simulink model "pmsm_foc_drive"  (R2026a)
settings: Solver=ode4  StopTime=5  FixedStep=1e-6
undefined symbols (not defined in the file): D, I_max, J, Ki_i, Ki_w, Kp_i, Kp_w, L, P, phi_m, Rs, T_s, Tpwm, V_max, Vdc
libraries: simulink x6, slpidlib x4, sl_discontinuities x1
settings Model: Creator=Lemão Som  LastModifiedBy=Lemão Som

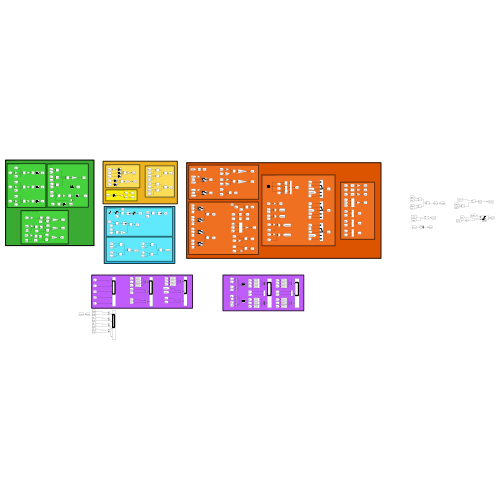
[thumbnail: Simulink's stored preview of the top-level diagram]
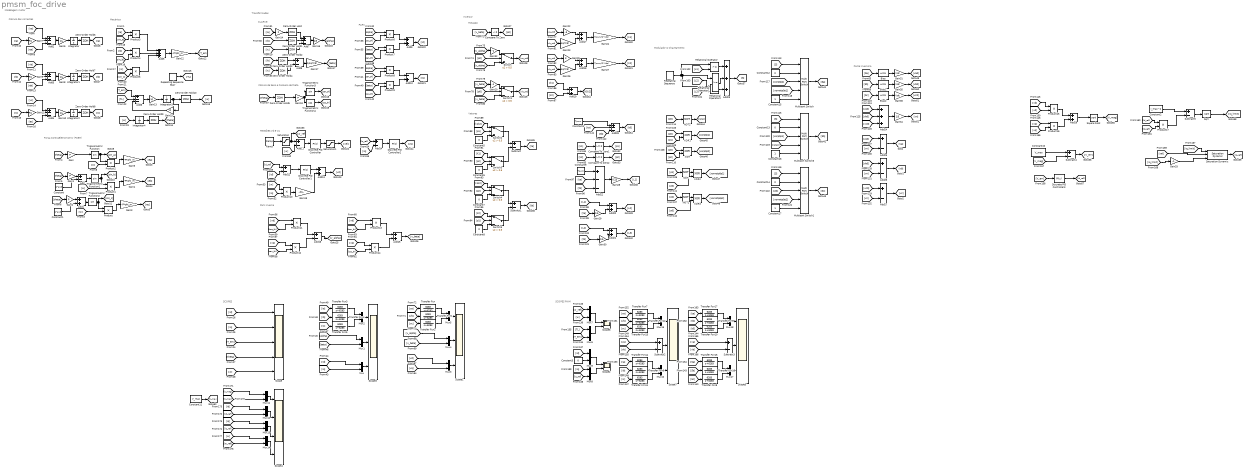
== system pmsm_foc_drive ==
  note: Ponte Inversora
  note: Modulador & Chaveamento
  note: Vetores
  note: Rotação
  note: SCOPES
  note: Cálculo de Seno e Cosseno de theta
  note: Transformadas
  note: Modelagem motor
  note: Inversor
  note: Park Inversa
  note: TENSÕES Vd E Vq
  note: PARK
  note: CLARKE
  note: Mecânica
  note: Força ContraEletromotriz (FCEM)
  note: Cálculo das correntes
  note: SCOPES PWM
  Add{,8,11..12,14,16,25..27} (9 alike) : Sum  Inputs=+-
  Add{1,9,13,15,17..21,29} (10 alike) : Sum
  Add10 : Sum  Inputs=-+
  Add{2..4,6..7,22,28} (7 alike) : Sum  Inputs=+--
  Add23 : Sum  Inputs=+++
  Add24 : Sum  Inputs=+++
  Add5 : Sum  Inputs=+++
  Bias : Bias  Bias=-0.5  SaturateOnIntegerOverflow=off
  Bias1 : Bias  Bias=-0.5  SaturateOnIntegerOverflow=off
  Bias2 : Bias  Bias=-0.5  SaturateOnIntegerOverflow=off
  Compare To Zero : simulink/Logic and Bit Operations/Compare To Zero  relop=<  OutDataTypeStr=boolean
  Compare To Zero1 : simulink/Logic and Bit Operations/Compare To Zero  relop=>=  OutDataTypeStr=boolean  ZeroCross=off
  Compare To Zero2 : simulink/Logic and Bit Operations/Compare To Zero  relop=>=  OutDataTypeStr=boolean  ZeroCross=off
  Constant : Constant  Value=2*pi/3
  Constant1 : Constant  Value=2*pi/3
  Constant10 : Constant  Value=V_max
  Constant11 : Constant  Value=V_max
  Constant{3,5..8,12..14} (8 alike) : Constant  Value=0
  Constant15 : Constant
  Constant16 : Constant
  Constant17 : Constant
  Constant2 : Constant  Value=I_max^2
  Constant4 : Constant  Value=Tpwm  VectorParams1D=off
  Constant9 : Constant  Value=Tpwm
  Discrete PID Controller : slpidlib/PID Controller  Controller=PI  Form=Parallel  TimeDomain=Discrete-time  UseExternalTs=off  SampleTime=T_s  IntegratorMethod=Forward Euler  FilterMethod=Forward Euler  ControllerParametersSource=internal  P=Kp_w  I=Ki_w  UseKiTs=off  D=0  UseExternalDerivativeSource=off  N=100  UseFilter=on  TunerSelectOption=Transfer Function Based (PID Tuner App)  InitialConditionSource=internal  InitialConditionForIntegrator=0  InitialConditionForFilter=0  DifferentiatorICPrevScaledInput=0  ExternalReset=none  TrackingMode=off  Kt=1  LimitOutput=on  SatLimitsSource=internal  UpperSaturationLimit=100  LowerSaturationLimit=-100  LinearizeAsGain=off  AntiWindupMode=clamping  Kb=1  LimitIntegrator=off  UpperIntegratorSaturationLimit=inf  LowerIntegratorSaturationLimit=-inf  POutMin=[]  POutMax=[]  IOutMin=[]  IOutMax=[]  DOutMin=[]  DOutMax=[]  NOutMin=[]  NOutMax=[]  SumOutMin=[]  SumOutMax=[]  SaturationOutMin=[]  SaturationOutMax=[]  PParamMin=[]  PParamMax=[]  IParamMin=[]  IParamMax=[]  DParamMin=[]  DParamMax=[]  NParamMin=[]  NParamMax=[]  KbParamMin=[]  KbParamMax=[]  KtParamMin=[]  KtParamMax=[]  KbOutMin=[]  KbOutMax=[]  KtOutMin=[]  KtOutMax=[]  IntegratorOutMin=[]  IntegratorOutMax=[]  FilterOutMin=[]  FilterOutMax=[]  SumI1OutMin=[]  SumI1OutMax=[]  SumI2OutMin=[]  SumI2OutMax=[]  SumI3OutMin=[]  SumI3OutMax=[]  SumI4OutMin=[]  SumI4OutMax=[]  SumDOutMin=[]  SumDOutMax=[]  DifferentiatorOutMin=[]  DifferentiatorOutMax=[]  FilterDiffOutCoefMin=[]  FilterDiffOutCoefMax=[]  ReciprocalOutMin=[]  ReciprocalOutMax=[]  SumDenOutMin=[]  SumDenOutMax=[]  SumNumOutMin=[]  SumNumOutMax=[]  DivideOutMin=[]  DivideOutMax=[]  UdiffTsProdOutMin=[]  UdiffTsProdOutMax=[]  NTsProdOutMin=[]  NTsProdOutMax=[]  UintegralTsProdOutMin=[]  UintegralTsProdOutMax=[]  UngainTsProdOutMin=[]  UngainTsProdOutMax=[]  ClampingZeroOutDataTypeStr=Inherit: Inherit via back propagation  ClampingZeroOutMin=[]  ClampingZeroOutMax=[]  FilterDenConstantOutDataTypeStr=Inherit: Inherit via back propagation  FilterDenConstantOutMin=[]  FilterDenConstantOutMax=[]  PCopyOutDataTypeStr=Inherit: Inherit via back propagation  PCopyOutMin=[]  PCopyOutMax=[]  NCopyOutDataTypeStr=Inherit: Inherit via back propagation  NCopyOutMin=[]  NCopyOutMax=[]  IntegratorContinuousStateAttributes=''  IntegratorStateMustResolveToSignalObject=off  IntegratorRTWStateStorageClass=Auto  FilterContinuousStateAttributes=''  FilterStateMustResolveToSignalObject=off  FilterRTWStateStorageClass=Auto  ParallelPVariant=InternalParameters  IdealPVariant=Disabled  IVariant=InternalParameters  DVariant=Disabled  IntegratorVariant=Discrete  SatVariant=Enabled  AWVariant=DiscClampingParallel  PCopyVariant=Disabled  TRVariant=Disabled  FdbkBlocksVariant=Forward  IdealPFdbkVariant=Disabled  SatFdbkVariant=Disabled  DerivativeFilterVariant=Disabled  NVariant=Disabled  NCopyVariant=Disabled_SignalSpec  FilterICVariant=Disabled  IntegratorICVariant=InternalICs  ExternalResetVariant=Disabled  TRSumVariant=Passthrough  SumFdbkVariant=Disabled  SumVariant=Sum_PI  TsampFilterVariant=InternalTs  TsampNgainVariant=Passthrough  TsampIntegralVariant=Disabled_SignalSpec  ExternalSaturationOutDataTypeStr=Inherit: Same as second input  DerivativeSourceVariant=Disabled  PreIntVariant=InternalPreInt
      settings: LibrarySourceBlock=simulink/Discrete/Discrete PID Controller
  Discrete PID Controller1 : slpidlib/PID Controller  Controller=PI  Form=Parallel  TimeDomain=Discrete-time  UseExternalTs=off  SampleTime=T_s  IntegratorMethod=Forward Euler  FilterMethod=Forward Euler  ControllerParametersSource=internal  P=Kp_i  I=Ki_i  UseKiTs=off  D=0  UseExternalDerivativeSource=off  N=100  UseFilter=on  TunerSelectOption=Transfer Function Based (PID Tuner App)  InitialConditionSource=internal  InitialConditionForIntegrator=0  InitialConditionForFilter=0  DifferentiatorICPrevScaledInput=0  ExternalReset=none  TrackingMode=off  Kt=1  LimitOutput=on  SatLimitsSource=internal  UpperSaturationLimit=V_max  LowerSaturationLimit=-V_max  LinearizeAsGain=off  AntiWindupMode=clamping  Kb=1  LimitIntegrator=off  UpperIntegratorSaturationLimit=inf  LowerIntegratorSaturationLimit=-inf  POutMin=[]  POutMax=[]  IOutMin=[]  IOutMax=[]  DOutMin=[]  DOutMax=[]  NOutMin=[]  NOutMax=[]  SumOutMin=[]  SumOutMax=[]  SaturationOutMin=[]  SaturationOutMax=[]  PParamMin=[]  PParamMax=[]  IParamMin=[]  IParamMax=[]  DParamMin=[]  DParamMax=[]  NParamMin=[]  NParamMax=[]  KbParamMin=[]  KbParamMax=[]  KtParamMin=[]  KtParamMax=[]  KbOutMin=[]  KbOutMax=[]  KtOutMin=[]  KtOutMax=[]  IntegratorOutMin=[]  IntegratorOutMax=[]  FilterOutMin=[]  FilterOutMax=[]  SumI1OutMin=[]  SumI1OutMax=[]  SumI2OutMin=[]  SumI2OutMax=[]  SumI3OutMin=[]  SumI3OutMax=[]  SumI4OutMin=[]  SumI4OutMax=[]  SumDOutMin=[]  SumDOutMax=[]  DifferentiatorOutMin=[]  DifferentiatorOutMax=[]  FilterDiffOutCoefMin=[]  FilterDiffOutCoefMax=[]  ReciprocalOutMin=[]  ReciprocalOutMax=[]  SumDenOutMin=[]  SumDenOutMax=[]  SumNumOutMin=[]  SumNumOutMax=[]  DivideOutMin=[]  DivideOutMax=[]  UdiffTsProdOutMin=[]  UdiffTsProdOutMax=[]  NTsProdOutMin=[]  NTsProdOutMax=[]  UintegralTsProdOutMin=[]  UintegralTsProdOutMax=[]  UngainTsProdOutMin=[]  UngainTsProdOutMax=[]  ClampingZeroOutDataTypeStr=Inherit: Inherit via back propagation  ClampingZeroOutMin=[]  ClampingZeroOutMax=[]  FilterDenConstantOutDataTypeStr=Inherit: Inherit via back propagation  FilterDenConstantOutMin=[]  FilterDenConstantOutMax=[]  PCopyOutDataTypeStr=Inherit: Inherit via back propagation  PCopyOutMin=[]  PCopyOutMax=[]  NCopyOutDataTypeStr=Inherit: Inherit via back propagation  NCopyOutMin=[]  NCopyOutMax=[]  IntegratorContinuousStateAttributes=''  IntegratorStateMustResolveToSignalObject=off  IntegratorRTWStateStorageClass=Auto  FilterContinuousStateAttributes=''  FilterStateMustResolveToSignalObject=off  FilterRTWStateStorageClass=Auto  ParallelPVariant=InternalParameters  IdealPVariant=Disabled  IVariant=InternalParameters  DVariant=Disabled  IntegratorVariant=Discrete  SatVariant=Enabled  AWVariant=DiscClampingParallel  PCopyVariant=Disabled  TRVariant=Disabled  FdbkBlocksVariant=Forward  IdealPFdbkVariant=Disabled  SatFdbkVariant=Disabled  DerivativeFilterVariant=Disabled  NVariant=Disabled  NCopyVariant=Disabled_SignalSpec  FilterICVariant=Disabled  IntegratorICVariant=InternalICs  ExternalResetVariant=Disabled  TRSumVariant=Passthrough  SumFdbkVariant=Disabled  SumVariant=Sum_PI  TsampFilterVariant=InternalTs  TsampNgainVariant=Passthrough  TsampIntegralVariant=Disabled_SignalSpec  ExternalSaturationOutDataTypeStr=Inherit: Same as second input  DerivativeSourceVariant=Disabled  PreIntVariant=InternalPreInt
      settings: LibrarySourceBlock=simulink/Discrete/Discrete PID Controller
  Discrete PID Controller2 : slpidlib/PID Controller  Controller=PI  Form=Parallel  TimeDomain=Discrete-time  UseExternalTs=off  SampleTime=T_s  IntegratorMethod=Forward Euler  FilterMethod=Forward Euler  ControllerParametersSource=internal  P=Kp_i  I=Ki_i  UseKiTs=off  D=0  UseExternalDerivativeSource=off  N=100  UseFilter=on  TunerSelectOption=Transfer Function Based (PID Tuner App)  InitialConditionSource=internal  InitialConditionForIntegrator=0  InitialConditionForFilter=0  DifferentiatorICPrevScaledInput=0  ExternalReset=none  TrackingMode=off  Kt=1  LimitOutput=on  SatLimitsSource=internal  UpperSaturationLimit=V_max  LowerSaturationLimit=-V_max  LinearizeAsGain=off  AntiWindupMode=clamping  Kb=1  LimitIntegrator=off  UpperIntegratorSaturationLimit=inf  LowerIntegratorSaturationLimit=-inf  POutMin=[]  POutMax=[]  IOutMin=[]  IOutMax=[]  DOutMin=[]  DOutMax=[]  NOutMin=[]  NOutMax=[]  SumOutMin=[]  SumOutMax=[]  SaturationOutMin=[]  SaturationOutMax=[]  PParamMin=[]  PParamMax=[]  IParamMin=[]  IParamMax=[]  DParamMin=[]  DParamMax=[]  NParamMin=[]  NParamMax=[]  KbParamMin=[]  KbParamMax=[]  KtParamMin=[]  KtParamMax=[]  KbOutMin=[]  KbOutMax=[]  KtOutMin=[]  KtOutMax=[]  IntegratorOutMin=[]  IntegratorOutMax=[]  FilterOutMin=[]  FilterOutMax=[]  SumI1OutMin=[]  SumI1OutMax=[]  SumI2OutMin=[]  SumI2OutMax=[]  SumI3OutMin=[]  SumI3OutMax=[]  SumI4OutMin=[]  SumI4OutMax=[]  SumDOutMin=[]  SumDOutMax=[]  DifferentiatorOutMin=[]  DifferentiatorOutMax=[]  FilterDiffOutCoefMin=[]  FilterDiffOutCoefMax=[]  ReciprocalOutMin=[]  ReciprocalOutMax=[]  SumDenOutMin=[]  SumDenOutMax=[]  SumNumOutMin=[]  SumNumOutMax=[]  DivideOutMin=[]  DivideOutMax=[]  UdiffTsProdOutMin=[]  UdiffTsProdOutMax=[]  NTsProdOutMin=[]  NTsProdOutMax=[]  UintegralTsProdOutMin=[]  UintegralTsProdOutMax=[]  UngainTsProdOutMin=[]  UngainTsProdOutMax=[]  ClampingZeroOutDataTypeStr=Inherit: Inherit via back propagation  ClampingZeroOutMin=[]  ClampingZeroOutMax=[]  FilterDenConstantOutDataTypeStr=Inherit: Inherit via back propagation  FilterDenConstantOutMin=[]  FilterDenConstantOutMax=[]  PCopyOutDataTypeStr=Inherit: Inherit via back propagation  PCopyOutMin=[]  PCopyOutMax=[]  NCopyOutDataTypeStr=Inherit: Inherit via back propagation  NCopyOutMin=[]  NCopyOutMax=[]  IntegratorContinuousStateAttributes=''  IntegratorStateMustResolveToSignalObject=off  IntegratorRTWStateStorageClass=Auto  FilterContinuousStateAttributes=''  FilterStateMustResolveToSignalObject=off  FilterRTWStateStorageClass=Auto  ParallelPVariant=InternalParameters  IdealPVariant=Disabled  IVariant=InternalParameters  DVariant=Disabled  IntegratorVariant=Discrete  SatVariant=Enabled  AWVariant=DiscClampingParallel  PCopyVariant=Disabled  TRVariant=Disabled  FdbkBlocksVariant=Forward  IdealPFdbkVariant=Disabled  SatFdbkVariant=Disabled  DerivativeFilterVariant=Disabled  NVariant=Disabled  NCopyVariant=Disabled_SignalSpec  FilterICVariant=Disabled  IntegratorICVariant=InternalICs  ExternalResetVariant=Disabled  TRSumVariant=Passthrough  SumFdbkVariant=Disabled  SumVariant=Sum_PI  TsampFilterVariant=InternalTs  TsampNgainVariant=Passthrough  TsampIntegralVariant=Disabled_SignalSpec  ExternalSaturationOutDataTypeStr=Inherit: Same as second input  DerivativeSourceVariant=Disabled  PreIntVariant=InternalPreInt
      settings: LibrarySourceBlock=simulink/Discrete/Discrete PID Controller
  Discrete PID Controller3 : slpidlib/PID Controller  Controller=PI  Form=Parallel  TimeDomain=Discrete-time  UseExternalTs=off  SampleTime=T_s  IntegratorMethod=Forward Euler  FilterMethod=Forward Euler  ControllerParametersSource=internal  P=0  I=5  UseKiTs=off  D=0  UseExternalDerivativeSource=off  N=100  UseFilter=on  TunerSelectOption=Transfer Function Based (PID Tuner App)  InitialConditionSource=internal  InitialConditionForIntegrator=0  InitialConditionForFilter=0  DifferentiatorICPrevScaledInput=0  ExternalReset=none  TrackingMode=off  Kt=1  LimitOutput=on  SatLimitsSource=internal  UpperSaturationLimit=0  LowerSaturationLimit=-100  LinearizeAsGain=off  AntiWindupMode=clamping  Kb=1  LimitIntegrator=off  UpperIntegratorSaturationLimit=inf  LowerIntegratorSaturationLimit=-inf  POutMin=[]  POutMax=[]  IOutMin=[]  IOutMax=[]  DOutMin=[]  DOutMax=[]  NOutMin=[]  NOutMax=[]  SumOutMin=[]  SumOutMax=[]  SaturationOutMin=[]  SaturationOutMax=[]  PParamMin=[]  PParamMax=[]  IParamMin=[]  IParamMax=[]  DParamMin=[]  DParamMax=[]  NParamMin=[]  NParamMax=[]  KbParamMin=[]  KbParamMax=[]  KtParamMin=[]  KtParamMax=[]  KbOutMin=[]  KbOutMax=[]  KtOutMin=[]  KtOutMax=[]  IntegratorOutMin=[]  IntegratorOutMax=[]  FilterOutMin=[]  FilterOutMax=[]  SumI1OutMin=[]  SumI1OutMax=[]  SumI2OutMin=[]  SumI2OutMax=[]  SumI3OutMin=[]  SumI3OutMax=[]  SumI4OutMin=[]  SumI4OutMax=[]  SumDOutMin=[]  SumDOutMax=[]  DifferentiatorOutMin=[]  DifferentiatorOutMax=[]  FilterDiffOutCoefMin=[]  FilterDiffOutCoefMax=[]  ReciprocalOutMin=[]  ReciprocalOutMax=[]  SumDenOutMin=[]  SumDenOutMax=[]  SumNumOutMin=[]  SumNumOutMax=[]  DivideOutMin=[]  DivideOutMax=[]  UdiffTsProdOutMin=[]  UdiffTsProdOutMax=[]  NTsProdOutMin=[]  NTsProdOutMax=[]  UintegralTsProdOutMin=[]  UintegralTsProdOutMax=[]  UngainTsProdOutMin=[]  UngainTsProdOutMax=[]  ClampingZeroOutDataTypeStr=Inherit: Inherit via back propagation  ClampingZeroOutMin=[]  ClampingZeroOutMax=[]  FilterDenConstantOutDataTypeStr=Inherit: Inherit via back propagation  FilterDenConstantOutMin=[]  FilterDenConstantOutMax=[]  PCopyOutDataTypeStr=Inherit: Inherit via back propagation  PCopyOutMin=[]  PCopyOutMax=[]  NCopyOutDataTypeStr=Inherit: Inherit via back propagation  NCopyOutMin=[]  NCopyOutMax=[]  IntegratorContinuousStateAttributes=''  IntegratorStateMustResolveToSignalObject=off  IntegratorRTWStateStorageClass=Auto  FilterContinuousStateAttributes=''  FilterStateMustResolveToSignalObject=off  FilterRTWStateStorageClass=Auto  ParallelPVariant=InternalParameters  IdealPVariant=Disabled  IVariant=InternalParameters  DVariant=Disabled  IntegratorVariant=Discrete  SatVariant=Enabled  AWVariant=DiscClampingParallel  PCopyVariant=Disabled  TRVariant=Disabled  FdbkBlocksVariant=Forward  IdealPFdbkVariant=Disabled  SatFdbkVariant=Disabled  DerivativeFilterVariant=Disabled  NVariant=Disabled  NCopyVariant=Disabled_SignalSpec  FilterICVariant=Disabled  IntegratorICVariant=InternalICs  ExternalResetVariant=Disabled  TRSumVariant=Passthrough  SumFdbkVariant=Disabled  SumVariant=Sum_PI  TsampFilterVariant=InternalTs  TsampNgainVariant=Passthrough  TsampIntegralVariant=Disabled_SignalSpec  ExternalSaturationOutDataTypeStr=Inherit: Same as second input  DerivativeSourceVariant=Disabled  PreIntVariant=InternalPreInt
      settings: LibrarySourceBlock=simulink/Discrete/Discrete PID Controller
  Gain{,1..2,18} (4 alike) : Gain  Gain=P
  Gain10 : Gain  Gain=1/L
  Gain11 : Gain  Gain=Rs
  Gain{3..5,12} (4 alike) : Gain  Gain=-P*phi_m
  Gain13 : Gain  Gain=1/J
  Gain14 : Gain  Gain=2
  Gain15 : Gain  Gain=D
  Gain16 : Gain  Gain=1/3
  Gain17 : Gain  Gain=1/sqrt(3)
  Gain19 : Gain  Gain=-P*L
  Gain20 : Gain  Gain=-1
  Gain22 : Gain  Gain=-3
  Gain23 : Gain  Gain=sqrt(3)
  Gain24 : Gain  Gain=Tpwm/(2*Vdc)
  Gain25 : Gain  Gain=3
  Gain26 : Gain  Gain=sqrt(3)
  Gain27 : Gain  Gain=Tpwm/(2*Vdc)
  Gain28 : Gain  Gain=0.25
  Gain29 : Gain  Gain=0.5
  Gain30 : Gain  Gain=0.5
  Gain31 : Gain  Gain=Vdc
  Gain32 : Gain  Gain=-1
  Gain33 : Gain  Gain=-1
  Gain34 : Gain  Gain=1/3
  Gain35 : Gain  Gain=Vdc
  Gain36 : Gain  Gain=Vdc
  Gain6 : Gain  Gain=1/L
  Gain7 : Gain  Gain=Rs
  Gain8 : Gain  Gain=1/L
  Gain9 : Gain  Gain=Rs
  Integrator{,1..4} (5 alike) : Integrator
  Multiport Switch : MultiPortSwitch  DataPortOrder=Zero-based contiguous  Inputs=4  zeroidx=on  SaturateOnIntegerOverflow=off  InputSameDT=off
  Multiport Switch1 : MultiPortSwitch  DataPortOrder=Zero-based contiguous  Inputs=4  zeroidx=on  SaturateOnIntegerOverflow=off  InputSameDT=off
  Multiport Switch3 : MultiPortSwitch  DataPortOrder=Zero-based contiguous  Inputs=4  zeroidx=on  SaturateOnIntegerOverflow=off  InputSameDT=off
  Mux{,1,3..4,6..9,11..14} (12 alike) : Mux  Inputs=2
  Mux{2,5,10,15,17..18} (6 alike) : Mux  Inputs=3
  NOT : Logic  Operator=NOT  IconShape=distinctive  AllPortsSameDT=off  OutDataTypeStr=boolean
  NOT1 : Logic  Operator=NOT  IconShape=distinctive  AllPortsSameDT=off  OutDataTypeStr=boolean
  NOT2 : Logic  Operator=NOT  IconShape=distinctive  AllPortsSameDT=off  OutDataTypeStr=boolean
  Product{,1..17} (18 alike) : Product
  Ramp : simulink/Sources/Ramp  slope=600  start=0  InitialOutput=0
  Relational Operator : RelationalOperator  OutDataTypeStr=boolean  ZeroCross=off  RndMeth=Simplest  InputSameDT=off
  Relational Operator1 : RelationalOperator  OutDataTypeStr=boolean  ZeroCross=off  RndMeth=Simplest  InputSameDT=off
  Relational Operator2 : RelationalOperator  OutDataTypeStr=boolean  ZeroCross=off  RndMeth=Simplest  InputSameDT=off
  Repeating Sequence : simulink/Sources/Repeating Sequence  rep_seq_t="[0,  Tpwm/2,  Tpwm]"  rep_seq_y="[0,  Tpwm/2,  0]"
  Repeating Sequence Stair : simulink/Sources/Repeating Sequence Stair  OutValues=[0, 0, 30, 60, 20, 0]  tsamp=1  OutMin=[]  OutMax=[]  OutDataTypeStr=double  OutputDataTypeScalingMode=double  OutDataType=fixdt(0,8)  ConRadixGroup=Best Precision: Vector-wise  OutScaling=2^-12
  Saturation : Saturate  UpperLimit=600  LowerLimit=0
  Saturation Dynamic : sl_discontinuities/Saturation Dynamic  OutMin=[]  OutMax=[]  OutDataTypeStr=Inherit: Same as second input  OutDataType=fixdt(1, 16)  OutScaling=2^-10  DoSatur=off
      settings: LibrarySourceBlock=|
      | simulink/Discontinuities/Saturation
      | Dynamic
  Saturation1 : Saturate  UpperLimit=250  LowerLimit=-250
  Scope : Scope  NumInputPorts=5
      settings: ActiveDisplayYMinimum=-2.0872010914501411  ActiveDisplayYMaximum=2.3051801873025868  DataLoggingMaxPoints=5000000
  Scope{1,3,5,7} (4 alike) : Scope  NumInputPorts=3
      Scope1 settings: ActiveDisplayYMinimum=-212.18215181352596  ActiveDisplayYMaximum=212.24523390642534  DataLoggingMaxPoints=5000000
      Scope3 settings: ActiveDisplayYMinimum=-83.179010116842434  ActiveDisplayYMaximum=76.308984109608033  DataLoggingMaxPoints=5000000  DataLoggingVariableName=ScopeData3
      Scope5 settings: ActiveDisplayYMinimum=-1.2478982513130638E-5  ActiveDisplayYMaximum=0.00011231084261817577  DataLoggingMaxPoints=5000000  DataLoggingVariableName=ScopeData5
      Scope7 settings: ActiveDisplayYMinimum=-211.2425122148619  ActiveDisplayYMaximum=211.22890816173023  DataLoggingMaxPoints=5000000  DataLoggingVariableName=ScopeData8
  Scope2 : Scope  NumInputPorts=2
      settings: ActiveDisplayYMinimum=-2.1802925303492819  ActiveDisplayYMaximum=2.5453264970639906  DataLoggingVariableName=ScopeData2
  Scope4 : Scope  NumInputPorts=4
      settings: ActiveDisplayYMinimum=-65.070663771160056  ActiveDisplayYMaximum=585.63597394044064  DataLoggingMaxPoints=5000000  DataLoggingVariableName=ScopeData4
  Scope6 : Scope  NumInputPorts=2
      settings: ActiveDisplayYMinimum=-38.402869037438151  ActiveDisplayYMaximum=345.62582133694343  DataLoggingVariableName=ScopeData6
  Sqrt : Sqrt
  Square Root : Sqrt
  Subtract{,1..5} (6 alike) : Sum  Inputs=+-
  Switch{,1..5} (6 alike) : Switch  Criteria=u2 > Threshold  Threshold=0.5  SaturateOnIntegerOverflow=off  InputSameDT=off
  Transfer Fcn{,1..17} (18 alike) : TransferFcn  Numerator=[6283]  Denominator=[1 6283]
  Trigonometric Function{,1..3} (4 alike) : Trigonometry
  Trigonometric Function4 : Trigonometry  Operator=cos
  XOR{,1..3} (4 alike) : Logic  Operator=XOR  IconShape=distinctive  AllPortsSameDT=off  OutDataTypeStr=boolean
  Zero-Order Hold{,1..5} (6 alike) : ZeroOrderHold  SampleTime=Tpwm
  Zero-Order Hold{6..10} (5 alike) : ZeroOrderHold  SampleTime=T_s
  wires:
  [theta] -> Gain/1
  Gain/1 -> Trigonometric Function/1
  [theta] -> Gain1/1
  Gain1/1 -> Add/1
  Constant/1 -> Add/2
  Add/1 -> Trigonometric Function1/1
  [theta] -> Gain2/1
  Gain2/1 -> Add1/1
  Add1/1 -> Trigonometric Function2/1
  Constant1/1 -> Add1/2
  Product/1 -> Gain3/1
  [w] -> Product/2
  Product1/1 -> Gain4/1
  [w] -> Product1/2
  Trigonometric Function1/1 -> [sin_b], Product1/1
  Product2/1 -> Gain5/1
  [w] -> Product2/2
  Trigonometric Function/1 -> Product2/1, [sin_a]
  Trigonometric Function2/1 -> [sin_c], Product/1
  Gain5/1 -> [ea]
  Gain4/1 -> [eb]
  Gain3/1 -> [ec]
  Add2/1 -> Gain6/1
  Add4/1 -> Gain10/1
  [ea] -> Add2/3
  [ec] -> Add4/3
  [ic] -> Gain11/1
  Add3/1 -> Gain8/1
  Gain11/1 -> Add4/2
  Gain6/1 -> Integrator/1
  Gain10/1 -> Integrator2/1
  Gain7/1 -> Add2/2
  [eb] -> Add3/3
  [vb] -> Add3/1
  [vc] -> Add4/1
  [ib] -> Gain9/1
  Gain8/1 -> Integrator1/1
  [ia] -> Gain7/1
  [va] -> Add2/1
  Gain9/1 -> Add3/2
  [ia] -> Product3/1
  [ib] -> Product4/1
  [ic] -> Product5/1
  [sin_a] -> Product3/2
  [sin_b] -> Product4/2
  [sin_c] -> Product5/2
  Product3/1 -> Add5/1
  Product4/1 -> Add5/2
  Product5/1 -> Add5/3
  Add5/1 -> Gain12/1
  Gain12/1 -> [T_em]
  [T_em] -> Add6/1
  [TL] -> Add6/2
  Add6/1 -> Gain13/1
  Gain13/1 -> Integrator3/1
  Integrator3/1 -> Gain15/1, Zero-Order Hold10/1
  [w] -> Integrator4/1
  Integrator4/1 -> Zero-Order Hold9/1
  Gain15/1 -> Add6/3
  Repeating Sequence Stair/1 -> [TL]
  [ic] -> Zero-Order Hold2/1
  [ib] -> Zero-Order Hold1/1
  [ia] -> Gain14/1
  Gain14/1 -> Zero-Order Hold/1
  Add7/1 -> Gain16/1
  Gain16/1 -> [alpha]
  [ib] -> Zero-Order Hold3/1
  [ic] -> Zero-Order Hold4/1
  Add8/1 -> Gain17/1
  Gain17/1 -> [beta]
  [theta] -> Zero-Order Hold5/1
  Gain18/1 -> Trigonometric Function4/1, Trigonometric Function3/1
  Trigonometric Function3/1 -> [sen_th]
  Trigonometric Function4/1 -> [cos_th]
  [alpha] -> Product6/1
  [cos_th] -> Product6/2
  [sen_th] -> Product7/2
  [beta] -> Product7/1
  Product6/1 -> Add9/1
  Product7/1 -> Add9/2
  Add9/1 -> [id]
  [sen_th] -> Product8/2
  Product8/1 -> Add10/1
  [beta] -> Product9/1
  Product9/1 -> Add10/2
  [cos_th] -> Product9/2
  Add10/1 -> [iq]
  [alpha] -> Product8/1
  Ramp/1 -> Saturation/1
  Saturation/1 -> Add11/1, [w_ref]
  [w] -> Add11/2
  Add11/1 -> Discrete PID Controller/1
  Discrete PID Controller/1 -> Saturation1/1
  Saturation1/1 -> [vel]
  [id_ref] -> Add12/1
  [id] -> Add12/2
  Discrete PID Controller1/1 -> Add13/1
  [iq] -> Product10/2
  [w] -> Product10/1
  Product10/1 -> Gain19/1
  Gain19/1 -> Add13/2
  Add13/1 -> [vd]
  [iq_ref] -> Add14/1
  [iq] -> Add14/2
  Add14/1 -> Discrete PID Controller2/1
  Discrete PID Controller2/1 -> [vq]
  [vd] -> Product11/1
  [cos_th] -> Product11/2
  [vq] -> Product12/1
  [sen_th] -> Product12/2
  Product11/1 -> Add16/1
  Product12/1 -> Add16/2
  Add16/1 -> [v_alpha]
  [sen_th] -> Product13/2
  [vd] -> Product13/1
  Add15/1 -> [v_beta]
  [vq] -> Product14/1
  Product13/1 -> Add15/1
  [cos_th] -> Product14/2
  Product14/1 -> Add15/2
  [w] -> Scope/5
  [theta] -> Scope/4
  [beta] -> Mux1/2
  [alpha] -> Mux1/1
  [v_beta] -> Compare To Zero/1
  Compare To Zero/1 -> [p0]
  [p0] -> Switch/2
  [v_alpha] -> Switch/3
  Switch/1 -> [va_rot]
  Switch1/1 -> [vb_rot]
  [p0] -> Switch1/2
  [v_beta] -> Switch1/3
  [va_rot] -> Gain22/1
  [vb_rot] -> Gain23/1
  Gain22/1 -> Add17/1
  Gain23/1 -> Add17/2
  Add17/1 -> Gain24/1
  Gain24/1 -> [k1]
  [va_rot] -> Gain25/1
  Gain25/1 -> Add18/1
  Gain27/1 -> [k2]
  [vb_rot] -> Gain26/1
  Gain26/1 -> Add18/2
  Add18/1 -> Gain27/1
  [k1] -> Compare To Zero1/1
  [k2] -> Compare To Zero2/1
  Compare To Zero1/1 -> [p1]
  Compare To Zero2/1 -> [p2]
  [k1] -> Add19/1
  [k2] -> Add19/2
  Add19/1 -> [k1k2]
  [p1] -> Switch2/2
  [k1k2] -> Switch2/1
  Constant5/1 -> Switch2/3
  [k1] -> Switch3/1
  [p2] -> Switch3/2
  Constant6/1 -> Switch3/3
  Switch2/1 -> Subtract/1
  Switch3/1 -> Subtract/2
  Subtract/1 -> [ta]
  [k2] -> Switch5/1
  Switch4/1 -> Subtract1/1
  [k1k2] -> Switch4/1
  [p2] -> Switch4/2
  Switch5/1 -> Subtract1/2
  Constant8/1 -> Switch5/3
  Constant7/1 -> Switch4/3
  Subtract1/1 -> [tb]
  [p1] -> Switch5/2
  Constant9/1 -> Add22/1
  [ta] -> Add22/2
  [tb] -> Add22/3
  Add22/1 -> Gain28/1
  Gain28/1 -> [L1]
  [L1] -> Add20/1
  [ta] -> Gain29/1
  Gain29/1 -> Add20/2
  Add20/1 -> [L2]
  [L2] -> Add21/1
  [tb] -> Gain30/1
  Gain30/1 -> Add21/2
  Add21/1 -> [L3]
  Repeating Sequence/1 -> Relational Operator1/1, Relational Operator2/1, Relational Operator/1
  [L1] -> Relational Operator/2
  [L2] -> Relational Operator2/2
  [L3] -> Relational Operator1/2
  Add23/1 -> [S]
  [p0] -> XOR/1
  [p2] -> XOR/2
  [p0] -> XOR1/1
  [p1] -> XOR1/2
  [p1] -> NOT/1
  NOT/1 -> XOR2/1
  [p0] -> XOR2/2
  NOT1/1 -> XOR3/1
  [p2] -> NOT1/1
  [p0] -> XOR3/2
  Multiport Switch/1 -> [Sa]
  [p0] -> NOT2/1
  NOT2/1 -> [notp0]
  [S] -> Multiport Switch/1
  Constant12/1 -> Multiport Switch/2
  XOR1/1 -> [xorp0p1]
  XOR/1 -> [xorp0p2]
  XOR3/1 -> [xornotp0p2]
  XOR2/1 -> [xornotp0p1]
  [xorp0p2] -> Multiport Switch/3
  [xornotp0p1] -> Multiport Switch/4
  Constant15/1 -> Multiport Switch/5
  Multiport Switch3/1 -> [Sb]
  [S] -> Multiport Switch3/1
  Constant13/1 -> Multiport Switch3/2
  Constant16/1 -> Multiport Switch3/5
  [notp0] -> Multiport Switch3/4
  [xorp0p1] -> Multiport Switch3/3
  Multiport Switch1/1 -> [Sc]
  [S] -> Multiport Switch1/1
  Constant14/1 -> Multiport Switch1/2
  Constant17/1 -> Multiport Switch1/5
  [xornotp0p2] -> Multiport Switch1/4
  [p0] -> Multiport Switch1/3
  [Sa] -> Bias/1
  [Sb] -> Bias1/1
  [Sc] -> Bias2/1
  [va0] -> Add24/1
  [vb0] -> Add24/2
  [vc0] -> Add24/3
  Add24/1 -> Gain34/1
  Gain34/1 -> [vn]
  Bias/1 -> Gain31/1
  Bias1/1 -> Gain35/1
  Gain35/1 -> [vb0]
  Gain31/1 -> [va0]
  Bias2/1 -> Gain36/1
  Gain36/1 -> [vc0]
  Zero-Order Hold/1 -> Add7/1
  Zero-Order Hold1/1 -> Add7/2
  Zero-Order Hold2/1 -> Add7/3
  Zero-Order Hold3/1 -> Add8/1
  Zero-Order Hold4/1 -> Add8/2
  [v_alpha] -> Gain32/1
  Gain32/1 -> Switch/1
  [v_beta] -> Gain20/1
  Gain20/1 -> Switch1/1
  Mux2/1 -> Scope3/1
  Mux1/1 -> Scope3/2
  Mux/1 -> Scope3/3
  Mux3/1 -> Scope1/3
  Mux4/1 -> Scope1/2
  Mux5/1 -> Scope1/1
  [va] -> Transfer Fcn/1
  [vb] -> Transfer Fcn1/1
  Transfer Fcn1/1 -> Mux5/2
  [vc] -> Transfer Fcn2/1
  Transfer Fcn2/1 -> Mux5/3
  Transfer Fcn/1 -> Mux5/1
  [ic] -> Transfer Fcn5/1
  [ia] -> Transfer Fcn3/1
  [ib] -> Transfer Fcn4/1
  Transfer Fcn3/1 -> Mux2/1
  Transfer Fcn4/1 -> Mux2/2
  Transfer Fcn5/1 -> Mux2/3
  [id] -> Scope/1
  [iq] -> Scope/2
  [T_em] -> Scope/3
  [v_alpha] -> Mux4/1
  [v_beta] -> Mux4/2
  [vd] -> Mux3/1
  [vq] -> Mux3/2
  [id] -> Mux/1
  [iq] -> Mux/2
  Zero-Order Hold5/1 -> Gain18/1
  Relational Operator2/1 -> Add23/2
  Relational Operator1/1 -> Add23/3
  Relational Operator/1 -> Add23/1
  Add25/1 -> [va]
  [vn] -> Add27/2
  [vb0] -> Add26/1
  [vn] -> Add25/2
  [vc0] -> Add27/1
  [va0] -> Add25/1
  Add26/1 -> [vb]
  Add27/1 -> [vc]
  [vn] -> Add26/2
  Mux7/1 -> Scope6/1
  [w] -> Mux7/2
  [w_ref] -> Mux7/1
  [T_em] -> Mux6/2
  [TL] -> Mux6/1
  Mux6/1 -> Scope6/2
  Constant3/1 -> Mux9/2
  [iq] -> Mux8/1
  Mux9/1 -> Scope2/1
  [id] -> Mux9/1
  Mux8/1 -> Scope2/2
  [vb] -> Subtract2/2
  [va] -> Transfer Fcn7/1
  Mux15/1 -> Scope7/1
  [vc] -> Transfer Fcn13/1
  Mux10/1 -> Scope7/3
  Transfer Fcn14/1 -> Mux10/1
  Transfer Fcn13/1 -> Mux15/3
  [ia] -> Transfer Fcn14/1
  Subtract2/1 -> Scope7/2
  Transfer Fcn11/1 -> Mux10/3
  [ic] -> Transfer Fcn11/1
  [ib] -> Transfer Fcn6/1
  Transfer Fcn6/1 -> Mux10/2
  Transfer Fcn12/1 -> Mux15/2
  [vb] -> Transfer Fcn12/1
  [va] -> Subtract2/1
  Transfer Fcn7/1 -> Mux15/1
  [iq_ref] -> Mux8/2
  Transfer Fcn17/1 -> Mux18/1
  [va] -> Subtract3/1
  [tb] -> Transfer Fcn9/1
  Transfer Fcn9/1 -> Mux18/2
  Transfer Fcn16/1 -> Mux17/2
  [Sb] -> Transfer Fcn16/1
  [Sc] -> Transfer Fcn8/1
  Transfer Fcn8/1 -> Mux17/3
  Subtract3/1 -> Scope5/2
  [Sa] -> Transfer Fcn15/1
  Transfer Fcn10/1 -> Mux18/3
  Transfer Fcn15/1 -> Mux17/1
  Mux17/1 -> Scope5/3
  [t0] -> Transfer Fcn10/1
  Mux18/1 -> Scope5/1
  [ta] -> Transfer Fcn17/1
  [vb] -> Subtract3/2
  Add28/1 -> [t0]
  [tb] -> Add28/3
  Constant4/1 -> Add28/1
  [ta] -> Add28/2
  Integrator/1 -> Zero-Order Hold6/1
  Zero-Order Hold6/1 -> [ia]
  Zero-Order Hold7/1 -> [ib]
  Integrator1/1 -> Zero-Order Hold7/1
  Integrator2/1 -> Zero-Order Hold8/1
  Zero-Order Hold8/1 -> [ic]
  Zero-Order Hold9/1 -> [theta]
  Zero-Order Hold10/1 -> [w]
  Add12/1 -> Discrete PID Controller1/1
  [vd] -> Product15/2
  [vd] -> Product15/1
  [vq] -> Product16/1
  [vq] -> Product16/2
  Product15/1 -> Add29/1
  Product16/1 -> Add29/2
  Add29/1 -> Square Root/1
  Square Root/1 -> [V_mag]
  Constant10/1 -> Subtract4/1
  [V_mag] -> Subtract4/2
  Subtract4/1 -> [V_err]
  [V_err] -> Discrete PID Controller3/1
  Discrete PID Controller3/1 -> [id_ref]
  [id_ref] -> Product17/1
  [id_ref] -> Product17/2
  Subtract5/1 -> Sqrt/1
  Sqrt/1 -> [iq_limit]
  [iq_limit] -> Saturation Dynamic/1
  [iq_limit] -> Gain33/1
  Gain33/1 -> Saturation Dynamic/3
  [vel] -> Saturation Dynamic/2
  Saturation Dynamic/1 -> [iq_ref]
  Product17/1 -> Subtract5/2
  Constant2/1 -> Subtract5/1
  Mux11/1 -> Scope4/1
  [V_mag] -> Mux11/1
  [V_max] -> Mux11/2
  [id_ref] -> Mux12/2
  [id] -> Mux12/1
  Mux12/1 -> Scope4/2
  [iq] -> Mux13/1
  [iq_ref] -> Mux13/2
  Mux13/1 -> Scope4/3
  [w_ref] -> Mux14/2
  [w] -> Mux14/1
  Mux14/1 -> Scope4/4
  Constant11/1 -> [V_max]
